simulink model "IEEE30_case"  (R2024b)
settings: Solver=FixedStepAuto  StartTime=0  StopTime=5  FixedStep=1e-7  RelTol=1e-3
values from neighbouring files (symbols this model uses):
  GFL_DFIG_7_C_bus = 0.08    [IEEE30_case_parameters.m]
  GFL_DFIG_7_D_mutual = 2.500000e+3    (= 2500)    [IEEE30_case_parameters.m]
  GFL_DFIG_7_f0 = 60    [IEEE30_case_parameters.m]
  GFL_DFIG_7_gPLLi = 3200    [IEEE30_case_parameters.m]
  GFL_DFIG_7_gPLLp = 650    [IEEE30_case_parameters.m]
  GFL_DFIG_7_H_WT = 0.4    [IEEE30_case_parameters.m]
  GFL_DFIG_7_Hg = 0.8    [IEEE30_case_parameters.m]
  GFL_DFIG_7_Igq_ref = 0    [IEEE30_case_parameters.m]
  GFL_DFIG_7_Ird_ref = 704.45696    [IEEE30_case_parameters.m]
  GFL_DFIG_7_KI_V = -300000    [IEEE30_case_parameters.m]
  GFL_DFIG_7_KP_V = -1000    [IEEE30_case_parameters.m]
  GFL_DFIG_7_Ksh = 1.254300e+4    (= 12543)    [IEEE30_case_parameters.m]
  GFL_DFIG_7_Lg = 0.000483    [IEEE30_case_parameters.m]
  GFL_DFIG_7_Lm_pu = 4    [IEEE30_case_parameters.m]
  GFL_DFIG_7_N = 100    [IEEE30_case_parameters.m]
  GFL_DFIG_7_p = 2    [IEEE30_case_parameters.m]
  GFL_DFIG_7_Pitch = 0    [IEEE30_case_parameters.m]
  GFL_DFIG_7_R = 44    [IEEE30_case_parameters.m]
  GFL_DFIG_7_Rg = 2.000000e-5    (= 2e-05)    [IEEE30_case_parameters.m]
  GFL_DFIG_7_rho = 1.225    [IEEE30_case_parameters.m]
  GFL_DFIG_7_rPLLi = 4500    [IEEE30_case_parameters.m]
  GFL_DFIG_7_rPLLp = 620    [IEEE30_case_parameters.m]
  GFL_DFIG_7_Rs_pu = 0.011    [IEEE30_case_parameters.m]
  GFL_DFIG_7_Sbase = 2.000000e+6    (= 2000000)    [IEEE30_case_parameters.m]
  GFL_DFIG_7_ugq_ref = 0    [IEEE30_case_parameters.m]
  GFL_DFIG_7_usd_ref = 0    [IEEE30_case_parameters.m]
  GFL_DFIG_7_Vbase = 690    [IEEE30_case_parameters.m]
  GFL_DFIG_7_Vdc_ref = 1200    [IEEE30_case_parameters.m]
  GFL_DFIG_7_wind = 12    [IEEE30_case_parameters.m]
  GFL_DFIG_7_wm_ref = 518.184209    [IEEE30_case_parameters.m]
  SG_D_13_D = 0.01056    [IEEE30_case_parameters.m]
  SG_D_13_EnableSaturation = 0    [IEEE30_case_parameters.m]
  SG_D_13_f0 = 60    [IEEE30_case_parameters.m]
  SG_D_13_H = 7.5    [IEEE30_case_parameters.m]
  SG_D_13_K_A = 20    [IEEE30_case_parameters.m]
  SG_D_13_K_E = 1.000000e+1    (= 10)    [IEEE30_case_parameters.m]
  SG_D_13_K_F = 2.363    [IEEE30_case_parameters.m]
  SG_D_13_K_s = 0.5    [IEEE30_case_parameters.m]
  SG_D_13_R_a = 0.001088    [IEEE30_case_parameters.m]
  SG_D_13_S_A = 1    [IEEE30_case_parameters.m]
  SG_D_13_S_B = 0.103    [IEEE30_case_parameters.m]
  SG_D_13_S_N = 10.659857    [IEEE30_case_parameters.m]
  SG_D_13_SpeedPara = 200    [IEEE30_case_parameters.m]
  SG_D_13_T_0 = 0.370163    [IEEE30_case_parameters.m]
  SG_D_13_T_1 = 0.3    [IEEE30_case_parameters.m]
  SG_D_13_T_2 = 0.05    [IEEE30_case_parameters.m]
  SG_D_13_T_3 = 0.02    [IEEE30_case_parameters.m]
  SG_D_13_T_4 = 0.005    [IEEE30_case_parameters.m]
  SG_D_13_T_A = 0.02    [IEEE30_case_parameters.m]
  SG_D_13_T_dd = 8.000000e+0    (= 8)    [IEEE30_case_parameters.m]
  SG_D_13_T_ddd = 0.04    [IEEE30_case_parameters.m]
  SG_D_13_T_E = 0.314    [IEEE30_case_parameters.m]
  SG_D_13_T_F = 0.35    [IEEE30_case_parameters.m]
  SG_D_13_T_qd = 0.8    [IEEE30_case_parameters.m]
  SG_D_13_T_qdd = 0.02    [IEEE30_case_parameters.m]
  SG_D_13_T_speed = 0.1    [IEEE30_case_parameters.m]
  SG_D_13_T_w = 0.5    [IEEE30_case_parameters.m]
  SG_D_13_V_ref = 1.696619    [IEEE30_case_parameters.m]
  SG_D_13_w_ref = 376.991118    [IEEE30_case_parameters.m]
  SG_D_13_x_d = 1.9    [IEEE30_case_parameters.m]
  SG_D_13_x_dd = 0.302    [IEEE30_case_parameters.m]
  SG_D_13_x_ddd = 0.204    [IEEE30_case_parameters.m]
  SG_D_13_x_l = 0.05    [IEEE30_case_parameters.m]
  SG_D_13_x_q = 1.3    [IEEE30_case_parameters.m]
  SG_D_13_x_qd = 0.5    [IEEE30_case_parameters.m]
  SG_D_13_x_qdd = 0.3    [IEEE30_case_parameters.m]
  SG_D_1_D = 0.01056    [IEEE30_case_parameters.m]
  SG_D_1_EnableSaturation = 0    [IEEE30_case_parameters.m]
  SG_D_1_f0 = 60    [IEEE30_case_parameters.m]
  SG_D_1_H = 7.5    [IEEE30_case_parameters.m]
  SG_D_1_K_A = 20    [IEEE30_case_parameters.m]
  SG_D_1_K_E = 1.000000e+1    (= 10)    [IEEE30_case_parameters.m]
  SG_D_1_K_F = 2.363    [IEEE30_case_parameters.m]
  SG_D_1_K_s = 0.5    [IEEE30_case_parameters.m]
  SG_D_1_R_a = 0.001088    [IEEE30_case_parameters.m]
  SG_D_1_S_A = 1    [IEEE30_case_parameters.m]
  SG_D_1_S_B = 0.103    [IEEE30_case_parameters.m]
  SG_D_1_S_N = 10.659857    [IEEE30_case_parameters.m]
  SG_D_1_SpeedPara = 200    [IEEE30_case_parameters.m]
  SG_D_1_T_0 = 0.259812    [IEEE30_case_parameters.m]
  SG_D_1_T_1 = 0.3    [IEEE30_case_parameters.m]
  SG_D_1_T_2 = 0.05    [IEEE30_case_parameters.m]
  SG_D_1_T_3 = 0.02    [IEEE30_case_parameters.m]
  SG_D_1_T_4 = 0.005    [IEEE30_case_parameters.m]
  SG_D_1_T_A = 0.02    [IEEE30_case_parameters.m]
  SG_D_1_T_dd = 8.000000e+0    (= 8)    [IEEE30_case_parameters.m]
  SG_D_1_T_ddd = 0.04    [IEEE30_case_parameters.m]
  SG_D_1_T_E = 0.314    [IEEE30_case_parameters.m]
  SG_D_1_T_F = 0.35    [IEEE30_case_parameters.m]
  SG_D_1_T_qd = 0.8    [IEEE30_case_parameters.m]
  SG_D_1_T_qdd = 0.02    [IEEE30_case_parameters.m]
  SG_D_1_T_speed = 0.1    [IEEE30_case_parameters.m]
  SG_D_1_T_w = 0.5    [IEEE30_case_parameters.m]
  SG_D_1_V_ref = 1.544107    [IEEE30_case_parameters.m]
  SG_D_1_w_ref = 376.991118    [IEEE30_case_parameters.m]
  SG_D_1_x_d = 1.9    [IEEE30_case_parameters.m]
  SG_D_1_x_dd = 0.302    [IEEE30_case_parameters.m]
  SG_D_1_x_ddd = 0.204    [IEEE30_case_parameters.m]
  SG_D_1_x_l = 0.05    [IEEE30_case_parameters.m]
  SG_D_1_x_q = 1.3    [IEEE30_case_parameters.m]
  SG_D_1_x_qd = 0.5    [IEEE30_case_parameters.m]
  SG_D_1_x_qdd = 0.3    [IEEE30_case_parameters.m]
  SG_D_22_D = 0.01056    [IEEE30_case_parameters.m]
  SG_D_22_EnableSaturation = 0    [IEEE30_case_parameters.m]
  SG_D_22_f0 = 60    [IEEE30_case_parameters.m]
  SG_D_22_H = 7.5    [IEEE30_case_parameters.m]
  SG_D_22_K_A = 20    [IEEE30_case_parameters.m]
  SG_D_22_K_E = 1.000000e+1    (= 10)    [IEEE30_case_parameters.m]
  SG_D_22_K_F = 2.363    [IEEE30_case_parameters.m]
  SG_D_22_K_s = 0.5    [IEEE30_case_parameters.m]
  SG_D_22_R_a = 0.001088    [IEEE30_case_parameters.m]
  SG_D_22_S_A = 1    [IEEE30_case_parameters.m]
  SG_D_22_S_B = 0.103    [IEEE30_case_parameters.m]
  SG_D_22_S_N = 10.659857    [IEEE30_case_parameters.m]
  SG_D_22_SpeedPara = 200    [IEEE30_case_parameters.m]
  SG_D_22_T_0 = 0.216121    [IEEE30_case_parameters.m]
  SG_D_22_T_1 = 0.3    [IEEE30_case_parameters.m]
  SG_D_22_T_2 = 0.05    [IEEE30_case_parameters.m]
  SG_D_22_T_3 = 0.02    [IEEE30_case_parameters.m]
  SG_D_22_T_4 = 0.005    [IEEE30_case_parameters.m]
  ... (+126 more)
(part 10 of 27)

== system IEEE30_case/AC_1/d_vq_bus_23_block ==
  note: d_vq_bus_23 in IEEE30_case
      | $37699111.8430775\,\mathrm{iq}_{\mathrm{bus},23}-376.991118430775\,\mathrm{vd}_{\mathrm{bus},23}$
      | Automatically generated on 2025-11-01 18:40:01 .
  Alge_iq_bus_23_4fd9f : Inport
  State_vd_bus_23_43c98 : Inport  Port=2
  Constant_376.991118430775_89ee7 : Constant  Value=376.991118430775
  Constant_37699111.8430775_5a930 : Constant  Value=37699111.8430775
  Product_5f7b2 : Product
  Product_6759d : Product
  Subtract_d8bec : Sum  Inputs=+-
  Blockout_d_vq_bus_23_b171c : Outport
  wires:
  Constant_37699111.8430775_5a930/1 -> Product_5f7b2/1
  Alge_iq_bus_23_4fd9f/1 -> Product_5f7b2/2
  Product_6759d/1 -> Subtract_d8bec/2
  State_vd_bus_23_43c98/1 -> Product_6759d/2
  Constant_376.991118430775_89ee7/1 -> Product_6759d/1
  Product_5f7b2/1 -> Subtract_d8bec/1
  Subtract_d8bec/1 -> Blockout_d_vq_bus_23_b171c/1

== system IEEE30_case/AC_1/d_vq_bus_24_block ==
  note: d_vq_bus_24 in IEEE30_case
      | $942477.796076938\,\mathrm{iq}_{\mathrm{bus},24}-376.991118430775\,\mathrm{vd}_{\mathrm{bus},24}$
      | Automatically generated on 2025-11-01 18:40:03 .
  Alge_iq_bus_24_0b825 : Inport
  State_vd_bus_24_b47e7 : Inport  Port=2
  Constant_376.991118430775_6b77a : Constant  Value=376.991118430775
  Constant_942477.796076938_b7520 : Constant  Value=942477.796076938
  Product_085e8 : Product
  Product_cc19f : Product
  Subtract_a05e3 : Sum  Inputs=+-
  Blockout_d_vq_bus_24_2859e : Outport
  wires:
  State_vd_bus_24_b47e7/1 -> Product_085e8/2
  Constant_942477.796076938_b7520/1 -> Product_cc19f/1
  Product_085e8/1 -> Subtract_a05e3/2
  Constant_376.991118430775_6b77a/1 -> Product_085e8/1
  Alge_iq_bus_24_0b825/1 -> Product_cc19f/2
  Product_cc19f/1 -> Subtract_a05e3/1
  Subtract_a05e3/1 -> Blockout_d_vq_bus_24_2859e/1

== system IEEE30_case/AC_1/d_vq_bus_25_block ==
  note: d_vq_bus_25 in IEEE30_case
      | $37699111.8430775\,\mathrm{iq}_{\mathrm{bus},25}-376.991118430775\,\mathrm{vd}_{\mathrm{bus},25}$
      | Automatically generated on 2025-11-01 18:40:05 .
  Alge_iq_bus_25_b52f0 : Inport
  State_vd_bus_25_5727a : Inport  Port=2
  Constant_376.991118430775_a3e2e : Constant  Value=376.991118430775
  Constant_37699111.8430775_b0c0a : Constant  Value=37699111.8430775
  Product_022ff : Product
  Product_2edfc : Product
  Subtract_ce7e6 : Sum  Inputs=+-
  Blockout_d_vq_bus_25_e403d : Outport
  wires:
  Alge_iq_bus_25_b52f0/1 -> Product_2edfc/2
  Constant_37699111.8430775_b0c0a/1 -> Product_2edfc/1
  Product_022ff/1 -> Subtract_ce7e6/2
  Constant_376.991118430775_a3e2e/1 -> Product_022ff/1
  State_vd_bus_25_5727a/1 -> Product_022ff/2
  Product_2edfc/1 -> Subtract_ce7e6/1
  Subtract_ce7e6/1 -> Blockout_d_vq_bus_25_e403d/1

== system IEEE30_case/AC_1/d_vq_bus_26_block ==
  note: d_vq_bus_26 in IEEE30_case
      | $37699111.8430775\,\mathrm{iq}_{\mathrm{bus},26}-376.991118430775\,\mathrm{vd}_{\mathrm{bus},26}$
      | Automatically generated on 2025-11-01 18:40:07 .
  Alge_iq_bus_26_172b0 : Inport
  State_vd_bus_26_21468 : Inport  Port=2
  Constant_376.991118430775_b7844 : Constant  Value=376.991118430775
  Constant_37699111.8430775_77cc8 : Constant  Value=37699111.8430775
  Product_15b09 : Product
  Product_a4d83 : Product
  Subtract_d1cbb : Sum  Inputs=+-
  Blockout_d_vq_bus_26_2e68a : Outport
  wires:
  Subtract_d1cbb/1 -> Blockout_d_vq_bus_26_2e68a/1
  Constant_37699111.8430775_77cc8/1 -> Product_a4d83/1
  Alge_iq_bus_26_172b0/1 -> Product_a4d83/2
  Constant_376.991118430775_b7844/1 -> Product_15b09/1
  Product_a4d83/1 -> Subtract_d1cbb/1
  State_vd_bus_26_21468/1 -> Product_15b09/2
  Product_15b09/1 -> Subtract_d1cbb/2

== system IEEE30_case/AC_1/d_vq_bus_27_block ==
  note: d_vq_bus_27 in IEEE30_case
      | $37699111.8430775\,\mathrm{iq}_{\mathrm{bus},27}-376.991118430775\,\mathrm{vd}_{\mathrm{bus},27}$
      | Automatically generated on 2025-11-01 18:40:08 .
  Alge_iq_bus_27_548e5 : Inport
  State_vd_bus_27_e355a : Inport  Port=2
  Constant_376.991118430775_3be52 : Constant  Value=376.991118430775
  Constant_37699111.8430775_fd80b : Constant  Value=37699111.8430775
  Product_a7865 : Product
  Product_b7592 : Product
  Subtract_05554 : Sum  Inputs=+-
  Blockout_d_vq_bus_27_9b6db : Outport
  wires:
  Subtract_05554/1 -> Blockout_d_vq_bus_27_9b6db/1
  Constant_37699111.8430775_fd80b/1 -> Product_b7592/1
  Alge_iq_bus_27_548e5/1 -> Product_b7592/2
  Product_a7865/1 -> Subtract_05554/2
  Constant_376.991118430775_3be52/1 -> Product_a7865/1
  Product_b7592/1 -> Subtract_05554/1
  State_vd_bus_27_e355a/1 -> Product_a7865/2

== system IEEE30_case/AC_1/d_vq_bus_28_block ==
  note: d_vq_bus_28 in IEEE30_case
      | $25132.7412287183\,\mathrm{iq}_{\mathrm{bus},28}-376.991118430775\,\mathrm{vd}_{\mathrm{bus},28}$
      | Automatically generated on 2025-11-01 18:40:10 .
  Alge_iq_bus_28_e3380 : Inport
  State_vd_bus_28_5e73c : Inport  Port=2
  Constant_25132.7412287183_edff6 : Constant  Value=25132.7412287183
  Constant_376.991118430775_78daa : Constant  Value=376.991118430775
  Product_1f4c4 : Product
  Product_9eeee : Product
  Subtract_e11d4 : Sum  Inputs=+-
  Blockout_d_vq_bus_28_fc78f : Outport
  wires:
  Constant_25132.7412287183_edff6/1 -> Product_1f4c4/1
  Alge_iq_bus_28_e3380/1 -> Product_1f4c4/2
  Product_9eeee/1 -> Subtract_e11d4/2
  Constant_376.991118430775_78daa/1 -> Product_9eeee/1
  Product_1f4c4/1 -> Subtract_e11d4/1
  State_vd_bus_28_5e73c/1 -> Product_9eeee/2
  Subtract_e11d4/1 -> Blockout_d_vq_bus_28_fc78f/1

== system IEEE30_case/AC_1/d_vq_bus_29_block ==
  note: d_vq_bus_29 in IEEE30_case
      | $37699111.8430775\,\mathrm{iq}_{\mathrm{bus},29}-376.991118430775\,\mathrm{vd}_{\mathrm{bus},29}$
      | Automatically generated on 2025-11-01 18:40:12 .
  Alge_iq_bus_29_a773e : Inport
  State_vd_bus_29_8221e : Inport  Port=2
  Constant_376.991118430775_ce99e : Constant  Value=376.991118430775
  Constant_37699111.8430775_7e507 : Constant  Value=37699111.8430775
  Product_4bf07 : Product
  Product_e159a : Product
  Subtract_59131 : Sum  Inputs=+-
  Blockout_d_vq_bus_29_9ca95 : Outport
  wires:
  Subtract_59131/1 -> Blockout_d_vq_bus_29_9ca95/1
  Constant_37699111.8430775_7e507/1 -> Product_4bf07/1
  Alge_iq_bus_29_a773e/1 -> Product_4bf07/2
  Product_e159a/1 -> Subtract_59131/2
  Constant_376.991118430775_ce99e/1 -> Product_e159a/1
  Product_4bf07/1 -> Subtract_59131/1
  State_vd_bus_29_8221e/1 -> Product_e159a/2

== system IEEE30_case/AC_1/d_vq_bus_2_block ==
  note: d_vq_bus_2 in IEEE30_case
      | $8377.58040957278\,\mathrm{iq}_{\mathrm{bus},2}-376.991118430775\,\mathrm{vd}_{\mathrm{bus},2}$
      | Automatically generated on 2025-11-01 18:39:26 .
  Alge_iq_bus_2_6cf64 : Inport
  State_vd_bus_2_c8ab9 : Inport  Port=2
  Constant_376.991118430775_774b2 : Constant  Value=376.991118430775
  Constant_8377.58040957278_cfb02 : Constant  Value=8377.58040957278
  Product_7f39e : Product
  Product_d1afe : Product
  Subtract_105ce : Sum  Inputs=+-
  Blockout_d_vq_bus_2_d5528 : Outport
  wires:
  Subtract_105ce/1 -> Blockout_d_vq_bus_2_d5528/1
  Constant_8377.58040957278_cfb02/1 -> Product_7f39e/1
  Alge_iq_bus_2_6cf64/1 -> Product_7f39e/2
  Constant_376.991118430775_774b2/1 -> Product_d1afe/1
  Product_7f39e/1 -> Subtract_105ce/1
  State_vd_bus_2_c8ab9/1 -> Product_d1afe/2
  Product_d1afe/1 -> Subtract_105ce/2

== system IEEE30_case/AC_1/d_vq_bus_30_block ==
  note: d_vq_bus_30 in IEEE30_case
      | $37699111.8430775\,\mathrm{iq}_{\mathrm{bus},30}-376.991118430775\,\mathrm{vd}_{\mathrm{bus},30}$
      | Automatically generated on 2025-11-01 18:40:13 .
  Alge_iq_bus_30_b84d2 : Inport
  State_vd_bus_30_536bd : Inport  Port=2
  Constant_376.991118430775_6c92f : Constant  Value=376.991118430775
  Constant_37699111.8430775_51ba2 : Constant  Value=37699111.8430775
  Product_8ec72 : Product
  Product_a9806 : Product
  Subtract_97059 : Sum  Inputs=+-
  Blockout_d_vq_bus_30_e3d22 : Outport
  wires:
  Subtract_97059/1 -> Blockout_d_vq_bus_30_e3d22/1
  Constant_37699111.8430775_51ba2/1 -> Product_a9806/1
  Alge_iq_bus_30_b84d2/1 -> Product_a9806/2
  Constant_376.991118430775_6c92f/1 -> Product_8ec72/1
  Product_a9806/1 -> Subtract_97059/1
  State_vd_bus_30_536bd/1 -> Product_8ec72/2
  Product_8ec72/1 -> Subtract_97059/2

== system IEEE30_case/AC_1/d_vq_bus_3_block ==
  note: d_vq_bus_3 in IEEE30_case
      | $37699.1118430775\,\mathrm{iq}_{\mathrm{bus},3}-376.991118430775\,\mathrm{vd}_{\mathrm{bus},3}$
      | Automatically generated on 2025-11-01 18:39:27 .
  Alge_iq_bus_3_cb5cd : Inport
  State_vd_bus_3_2475d : Inport  Port=2
  Constant_376.991118430775_40eb7 : Constant  Value=376.991118430775
  Constant_37699.1118430775_dedd8 : Constant  Value=37699.1118430775
  Product_a5528 : Product
  Product_bea63 : Product
  Subtract_577e7 : Sum  Inputs=+-
  Blockout_d_vq_bus_3_10f19 : Outport
  wires:
  Subtract_577e7/1 -> Blockout_d_vq_bus_3_10f19/1
  Constant_37699.1118430775_dedd8/1 -> Product_a5528/1
  Alge_iq_bus_3_cb5cd/1 -> Product_a5528/2
  Product_bea63/1 -> Subtract_577e7/2
  Constant_376.991118430775_40eb7/1 -> Product_bea63/1
  Product_a5528/1 -> Subtract_577e7/1
  State_vd_bus_3_2475d/1 -> Product_bea63/2

== system IEEE30_case/AC_1/d_vq_bus_4_block ==
  note: d_vq_bus_4 in IEEE30_case
      | $37699.1118430775\,\mathrm{iq}_{\mathrm{bus},4}-376.991118430775\,\mathrm{vd}_{\mathrm{bus},4}$
      | Automatically generated on 2025-11-01 18:39:29 .
  Alge_iq_bus_4_edea5 : Inport
  State_vd_bus_4_783ad : Inport  Port=2
  Constant_376.991118430775_7c085 : Constant  Value=376.991118430775
  Constant_37699.1118430775_1ff83 : Constant  Value=37699.1118430775
  Product_afb80 : Product
  Product_bbdae : Product
  Subtract_ff271 : Sum  Inputs=+-
  Blockout_d_vq_bus_4_757f0 : Outport
  wires:
  Constant_37699.1118430775_1ff83/1 -> Product_afb80/1
  Alge_iq_bus_4_edea5/1 -> Product_afb80/2
  Product_bbdae/1 -> Subtract_ff271/2
  Constant_376.991118430775_7c085/1 -> Product_bbdae/1
  Product_afb80/1 -> Subtract_ff271/1
  State_vd_bus_4_783ad/1 -> Product_bbdae/2
  Subtract_ff271/1 -> Blockout_d_vq_bus_4_757f0/1

== system IEEE30_case/AC_1/d_vq_bus_5_block ==
  note: d_vq_bus_5 in IEEE30_case
      | $22307.1667710518\,\mathrm{iq}_{\mathrm{bus},5}-376.991118430775\,\mathrm{vd}_{\mathrm{bus},5}$
      | Automatically generated on 2025-11-01 18:39:31 .
  Alge_iq_bus_5_20adf : Inport
  State_vd_bus_5_28f77 : Inport  Port=2
  Constant_22307.1667710518_b913d : Constant  Value=22307.1667710518
  Constant_376.991118430775_7861f : Constant  Value=376.991118430775
  Product_25fa6 : Product
  Product_cf06c : Product
  Subtract_2168d : Sum  Inputs=+-
  Blockout_d_vq_bus_5_f1f0c : Outport
  wires:
  Constant_22307.1667710518_b913d/1 -> Product_25fa6/1
  Product_cf06c/1 -> Subtract_2168d/2
  Constant_376.991118430775_7861f/1 -> Product_cf06c/1
  Alge_iq_bus_5_20adf/1 -> Product_25fa6/2
  State_vd_bus_5_28f77/1 -> Product_cf06c/2
  Product_25fa6/1 -> Subtract_2168d/1
  Subtract_2168d/1 -> Blockout_d_vq_bus_5_f1f0c/1

== system IEEE30_case/AC_1/d_vq_bus_6_block ==
  note: d_vq_bus_6 in IEEE30_case
      | $18849.5559215388\,\mathrm{iq}_{\mathrm{bus},6}-376.991118430775\,\mathrm{vd}_{\mathrm{bus},6}$
      | Automatically generated on 2025-11-01 18:39:32 .
  Alge_iq_bus_6_8f458 : Inport
  State_vd_bus_6_1a151 : Inport  Port=2
  Constant_18849.5559215388_854b2 : Constant  Value=18849.5559215388
  Constant_376.991118430775_77bfe : Constant  Value=376.991118430775
  Product_ad02e : Product
  Product_e2853 : Product
  Subtract_ccaa3 : Sum  Inputs=+-
  Blockout_d_vq_bus_6_ac6cf : Outport
  wires:
  Constant_18849.5559215388_854b2/1 -> Product_ad02e/1
  Product_e2853/1 -> Subtract_ccaa3/2
  Alge_iq_bus_6_8f458/1 -> Product_ad02e/2
  Constant_376.991118430775_77bfe/1 -> Product_e2853/1
  State_vd_bus_6_1a151/1 -> Product_e2853/2
  Product_ad02e/1 -> Subtract_ccaa3/1
  Subtract_ccaa3/1 -> Blockout_d_vq_bus_6_ac6cf/1

== system IEEE30_case/AC_1/d_vq_bus_7_block ==
  note: d_vq_bus_7 in IEEE30_case
      | $37699.1118430775\,\mathrm{iq}_{\mathrm{bus},7}-376.991118430775\,\mathrm{vd}_{\mathrm{bus},7}$
      | Automatically generated on 2025-11-01 18:39:34 .
  Alge_iq_bus_7_86528 : Inport
  State_vd_bus_7_0bd1f : Inport  Port=2
  Constant_376.991118430775_95f94 : Constant  Value=376.991118430775
  Constant_37699.1118430775_46c75 : Constant  Value=37699.1118430775
  Product_8c587 : Product
  Product_cc660 : Product
  Subtract_38f8c : Sum  Inputs=+-
  Blockout_d_vq_bus_7_71b97 : Outport
  wires:
  Subtract_38f8c/1 -> Blockout_d_vq_bus_7_71b97/1
  Constant_37699.1118430775_46c75/1 -> Product_cc660/1
  Alge_iq_bus_7_86528/1 -> Product_cc660/2
  Product_8c587/1 -> Subtract_38f8c/2
  Constant_376.991118430775_95f94/1 -> Product_8c587/1
  Product_cc660/1 -> Subtract_38f8c/1
  State_vd_bus_7_0bd1f/1 -> Product_8c587/2

== system IEEE30_case/AC_1/d_vq_bus_8_block ==
  note: d_vq_bus_8 in IEEE30_case
      | $37699.1118430775\,\mathrm{iq}_{\mathrm{bus},8}-376.991118430775\,\mathrm{vd}_{\mathrm{bus},8}$
      | Automatically generated on 2025-11-01 18:39:36 .
  Alge_iq_bus_8_bb8a6 : Inport
  State_vd_bus_8_8cd22 : Inport  Port=2
  Constant_376.991118430775_aa994 : Constant  Value=376.991118430775
  Constant_37699.1118430775_3c9b2 : Constant  Value=37699.1118430775
  Product_1950e : Product
  Product_8773e : Product
  Subtract_0dd82 : Sum  Inputs=+-
  Blockout_d_vq_bus_8_7917f : Outport
  wires:
  Constant_37699.1118430775_3c9b2/1 -> Product_1950e/1
  Alge_iq_bus_8_bb8a6/1 -> Product_1950e/2
  Product_8773e/1 -> Subtract_0dd82/2
  Constant_376.991118430775_aa994/1 -> Product_8773e/1
  Product_1950e/1 -> Subtract_0dd82/1
  State_vd_bus_8_8cd22/1 -> Product_8773e/2
  Subtract_0dd82/1 -> Blockout_d_vq_bus_8_7917f/1

== system IEEE30_case/AC_1/d_vq_bus_9_block ==
  note: d_vq_bus_9 in IEEE30_case
      | $37699111.8430775\,\mathrm{iq}_{\mathrm{bus},9}-376.991118430775\,\mathrm{vd}_{\mathrm{bus},9}$
      | Automatically generated on 2025-11-01 18:39:37 .
  Alge_iq_bus_9_8054c : Inport
  State_vd_bus_9_08774 : Inport  Port=2
  Constant_376.991118430775_3b7d3 : Constant  Value=376.991118430775
  Constant_37699111.8430775_a1b9d : Constant  Value=37699111.8430775
  Product_85a06 : Product
  Product_e292a : Product
  Subtract_b525b : Sum  Inputs=+-
  Blockout_d_vq_bus_9_087a9 : Outport
  wires:
  Subtract_b525b/1 -> Blockout_d_vq_bus_9_087a9/1
  Constant_37699111.8430775_a1b9d/1 -> Product_e292a/1
  Alge_iq_bus_9_8054c/1 -> Product_e292a/2
  Product_85a06/1 -> Subtract_b525b/2
  Constant_376.991118430775_3b7d3/1 -> Product_85a06/1
  Product_e292a/1 -> Subtract_b525b/1
  State_vd_bus_9_08774/1 -> Product_85a06/2

== system IEEE30_case/AC_1/id_bus_10_block ==
  note: id_bus_10 in IEEE30_case
      | $\mathrm{id}_{\mathrm{line},6,10}-\mathrm{id}_{\mathrm{load},10}+\mathrm{id}_{\mathrm{line},9,10}-\mathrm{id}_{\mathrm{line},10,17}-\mathrm{id}_{\mathrm{line},10,20}-\mathrm{id}_{\mathrm{line},10,21}-\mathrm{id}_{\mathrm{line},10,22}$
      | Automatically generated on 2025-11-01 18:42:51 .
  State_id_load_10_705f8 : Inport
  State_id_line_6_10_65dc9 : Inport  Port=2
  State_id_line_9_10_7013c : Inport  Port=3
  State_id_line_10_17_ef9ff : Inport  Port=4
  State_id_line_10_20_18f02 : Inport  Port=5
  State_id_line_10_21_c8fce : Inport  Port=6
  State_id_line_10_22_301e1 : Inport  Port=7
  Add_81d1d : Sum
  Add_d7f77 : Sum
  Constant_-1_c0d8a : Constant  Value=-1
  Product_b469d : Product
  Subtract_5d409 : Sum  Inputs=+-
  Subtract_9e640 : Sum  Inputs=+-
  Subtract_a236b : Sum  Inputs=+-
  Subtract_d925d : Sum  Inputs=+-
  Blockout_id_bus_10_f7cfc : Outport
  wires:
  Constant_-1_c0d8a/1 -> Product_b469d/1
  Product_b469d/1 -> Add_d7f77/1
  Add_d7f77/1 -> Add_81d1d/1
  Add_81d1d/1 -> Subtract_a236b/1
  State_id_load_10_705f8/1 -> Product_b469d/2
  State_id_line_6_10_65dc9/1 -> Add_d7f77/2
  State_id_line_10_17_ef9ff/1 -> Subtract_a236b/2
  State_id_line_9_10_7013c/1 -> Add_81d1d/2
  Subtract_5d409/1 -> Subtract_d925d/1
  Subtract_a236b/1 -> Subtract_5d409/1
  State_id_line_10_20_18f02/1 -> Subtract_5d409/2
  State_id_line_10_21_c8fce/1 -> Subtract_d925d/2
  State_id_line_10_22_301e1/1 -> Subtract_9e640/2
  Subtract_d925d/1 -> Subtract_9e640/1
  Subtract_9e640/1 -> Blockout_id_bus_10_f7cfc/1

== system IEEE30_case/AC_1/id_bus_11_block ==
  note: id_bus_11 in IEEE30_case
      | $\mathrm{id}_{\mathrm{line},9,11}$
      | Automatically generated on 2025-11-01 18:42:52 .
  State_id_line_9_11_37f59 : Inport
  Blockout_id_bus_11_04e0f : Outport
  wires:
  State_id_line_9_11_37f59/1 -> Blockout_id_bus_11_04e0f/1

== system IEEE30_case/AC_1/id_bus_12_block ==
  note: id_bus_12 in IEEE30_case
      | $\mathrm{id}_{\mathrm{line},4,12}-\mathrm{id}_{\mathrm{load},12}-\mathrm{id}_{\mathrm{line},12,13}-\mathrm{id}_{\mathrm{line},12,14}-\mathrm{id}_{\mathrm{line},12,15}-\mathrm{id}_{\mathrm{line},12,16}$
      | Automatically generated on 2025-11-01 18:42:54 .
  State_id_load_12_8eb9c : Inport
  State_id_line_4_12_8182e : Inport  Port=2
  State_id_line_12_13_02bcf : Inport  Port=3
  State_id_line_12_14_017fa : Inport  Port=4
  State_id_line_12_15_e30db : Inport  Port=5
  State_id_line_12_16_2f396 : Inport  Port=6
  Add_340d6 : Sum
  Constant_-1_6c20b : Constant  Value=-1
  Product_d81ab : Product
  Subtract_4b682 : Sum  Inputs=+-
  Subtract_956ec : Sum  Inputs=+-
  Subtract_d4719 : Sum  Inputs=+-
  Subtract_d9b2f : Sum  Inputs=+-
  Blockout_id_bus_12_a7f7d : Outport
  wires:
  Constant_-1_6c20b/1 -> Product_d81ab/1
  Product_d81ab/1 -> Add_340d6/1
  Add_340d6/1 -> Subtract_956ec/1
  State_id_line_4_12_8182e/1 -> Add_340d6/2
  State_id_load_12_8eb9c/1 -> Product_d81ab/2
  Subtract_4b682/1 -> Subtract_d4719/1
  Subtract_956ec/1 -> Subtract_4b682/1
  State_id_line_12_13_02bcf/1 -> Subtract_956ec/2
  State_id_line_12_14_017fa/1 -> Subtract_4b682/2
  State_id_line_12_15_e30db/1 -> Subtract_d4719/2
  Subtract_d4719/1 -> Subtract_d9b2f/1
  State_id_line_12_16_2f396/1 -> Subtract_d9b2f/2
  Subtract_d9b2f/1 -> Blockout_id_bus_12_a7f7d/1

== system IEEE30_case/AC_1/id_bus_13_block ==
  note: id_bus_13 in IEEE30_case
      | $\mathrm{id}_{\mathrm{SG},D,13}+\mathrm{id}_{\mathrm{line},12,13}$
      | Automatically generated on 2025-11-01 18:42:57 .
  Input_id_SG_D_13_a3cac : Inport
  State_id_line_12_13_e1ea8 : Inport  Port=2
  Add_1f282 : Sum
  Blockout_id_bus_13_e8139 : Outport
  wires:
  Add_1f282/1 -> Blockout_id_bus_13_e8139/1
  State_id_line_12_13_e1ea8/1 -> Add_1f282/2
  Input_id_SG_D_13_a3cac/1 -> Add_1f282/1

== system IEEE30_case/AC_1/id_bus_14_block ==
  note: id_bus_14 in IEEE30_case
      | $\mathrm{id}_{\mathrm{line},12,14}-\mathrm{id}_{\mathrm{load},14}-\mathrm{id}_{\mathrm{line},14,15}$
      | Automatically generated on 2025-11-01 18:42:58 .
  State_id_load_14_8acb6 : Inport
  State_id_line_12_14_e86dc : Inport  Port=2
  State_id_line_14_15_8760d : Inport  Port=3
  Add_4b372 : Sum
  Constant_-1_29924 : Constant  Value=-1
  Product_0535b : Product
  Subtract_f026d : Sum  Inputs=+-
  Blockout_id_bus_14_a7723 : Outport
  wires:
  Product_0535b/1 -> Add_4b372/1
  Constant_-1_29924/1 -> Product_0535b/1
  Add_4b372/1 -> Subtract_f026d/1
  State_id_line_12_14_e86dc/1 -> Add_4b372/2
  State_id_load_14_8acb6/1 -> Product_0535b/2
  State_id_line_14_15_8760d/1 -> Subtract_f026d/2
  Subtract_f026d/1 -> Blockout_id_bus_14_a7723/1

== system IEEE30_case/AC_1/id_bus_15_block ==
  note: id_bus_15 in IEEE30_case
      | $\mathrm{id}_{\mathrm{line},12,15}-\mathrm{id}_{\mathrm{load},15}+\mathrm{id}_{\mathrm{line},14,15}-\mathrm{id}_{\mathrm{line},15,18}-\mathrm{id}_{\mathrm{line},15,23}$
      | Automatically generated on 2025-11-01 18:43:00 .
  State_id_load_15_060ab : Inport
  State_id_line_12_15_8e417 : Inport  Port=2
  State_id_line_14_15_22f97 : Inport  Port=3
  State_id_line_15_18_9837d : Inport  Port=4
  State_id_line_15_23_df0bc : Inport  Port=5
  Add_c531c : Sum
  Add_d2721 : Sum
  Constant_-1_33c67 : Constant  Value=-1
  Product_a587d : Product
  Subtract_6212d : Sum  Inputs=+-
  Subtract_7f898 : Sum  Inputs=+-
  Blockout_id_bus_15_03e1f : Outport
  wires:
  Constant_-1_33c67/1 -> Product_a587d/1
  Product_a587d/1 -> Add_c531c/1
  State_id_line_12_15_8e417/1 -> Add_c531c/2
  State_id_load_15_060ab/1 -> Product_a587d/2
  Add_c531c/1 -> Add_d2721/1
  Add_d2721/1 -> Subtract_6212d/1
  State_id_line_15_18_9837d/1 -> Subtract_6212d/2
  State_id_line_14_15_22f97/1 -> Add_d2721/2
  Subtract_6212d/1 -> Subtract_7f898/1
  State_id_line_15_23_df0bc/1 -> Subtract_7f898/2
  Subtract_7f898/1 -> Blockout_id_bus_15_03e1f/1

== system IEEE30_case/AC_1/id_bus_16_block ==
  note: id_bus_16 in IEEE30_case
      | $\mathrm{id}_{\mathrm{line},12,16}-\mathrm{id}_{\mathrm{load},16}-\mathrm{id}_{\mathrm{line},16,17}$
      | Automatically generated on 2025-11-01 18:43:02 .
  State_id_load_16_85ef4 : Inport
  State_id_line_12_16_31af9 : Inport  Port=2
  State_id_line_16_17_d7b9d : Inport  Port=3
  Add_c2788 : Sum
  Constant_-1_e4b07 : Constant  Value=-1
  Product_aea95 : Product
  Subtract_c106b : Sum  Inputs=+-
  Blockout_id_bus_16_3e58c : Outport
  wires:
  Constant_-1_e4b07/1 -> Product_aea95/1
  State_id_line_12_16_31af9/1 -> Add_c2788/2
  State_id_load_16_85ef4/1 -> Product_aea95/2
  Product_aea95/1 -> Add_c2788/1
  Subtract_c106b/1 -> Blockout_id_bus_16_3e58c/1
  Add_c2788/1 -> Subtract_c106b/1
  State_id_line_16_17_d7b9d/1 -> Subtract_c106b/2

== system IEEE30_case/AC_1/id_bus_17_block ==
  note: id_bus_17 in IEEE30_case
      | $\mathrm{id}_{\mathrm{line},10,17}-\mathrm{id}_{\mathrm{load},17}+\mathrm{id}_{\mathrm{line},16,17}$
      | Automatically generated on 2025-11-01 18:43:04 .
  State_id_load_17_98f31 : Inport
  State_id_line_10_17_3b6f4 : Inport  Port=2
  State_id_line_16_17_e2e89 : Inport  Port=3
  Add_4d1b5 : Sum
  Add_d5a9b : Sum
  Constant_-1_d3cb0 : Constant  Value=-1
  Product_e65a9 : Product
  Blockout_id_bus_17_5f54e : Outport
  wires:
  Product_e65a9/1 -> Add_d5a9b/1
  Constant_-1_d3cb0/1 -> Product_e65a9/1
  Add_d5a9b/1 -> Add_4d1b5/1
  State_id_line_10_17_3b6f4/1 -> Add_d5a9b/2
  State_id_load_17_98f31/1 -> Product_e65a9/2
  State_id_line_16_17_e2e89/1 -> Add_4d1b5/2
  Add_4d1b5/1 -> Blockout_id_bus_17_5f54e/1

== system IEEE30_case/AC_1/id_bus_18_block ==
  note: id_bus_18 in IEEE30_case
      | $\mathrm{id}_{\mathrm{line},15,18}-\mathrm{id}_{\mathrm{load},18}-\mathrm{id}_{\mathrm{line},18,19}$
      | Automatically generated on 2025-11-01 18:43:05 .
  State_id_load_18_b6089 : Inport
  State_id_line_15_18_185de : Inport  Port=2
  State_id_line_18_19_1fd25 : Inport  Port=3
  Add_02070 : Sum
  Constant_-1_09ca4 : Constant  Value=-1
  Product_47eef : Product
  Subtract_a4093 : Sum  Inputs=+-
  Blockout_id_bus_18_f6aba : Outport
  wires:
  Subtract_a4093/1 -> Blockout_id_bus_18_f6aba/1
  Product_47eef/1 -> Add_02070/1
  Constant_-1_09ca4/1 -> Product_47eef/1
  State_id_load_18_b6089/1 -> Product_47eef/2
  Add_02070/1 -> Subtract_a4093/1
  State_id_line_15_18_185de/1 -> Add_02070/2
  State_id_line_18_19_1fd25/1 -> Subtract_a4093/2

== system IEEE30_case/AC_1/id_bus_19_block ==
  note: id_bus_19 in IEEE30_case
      | $\mathrm{id}_{\mathrm{line},18,19}-\mathrm{id}_{\mathrm{load},19}-\mathrm{id}_{\mathrm{line},19,20}$
      | Automatically generated on 2025-11-01 18:43:07 .
  State_id_load_19_6dd0b : Inport
  State_id_line_18_19_4e3a3 : Inport  Port=2
  State_id_line_19_20_f791c : Inport  Port=3
  Add_1b5aa : Sum
  Constant_-1_3ab29 : Constant  Value=-1
  Product_b6dd6 : Product
  Subtract_f828e : Sum  Inputs=+-
  Blockout_id_bus_19_c959d : Outport
  wires:
  State_id_line_19_20_f791c/1 -> Subtract_f828e/2
  State_id_line_18_19_4e3a3/1 -> Add_1b5aa/2
  Constant_-1_3ab29/1 -> Product_b6dd6/1
  State_id_load_19_6dd0b/1 -> Product_b6dd6/2
  Product_b6dd6/1 -> Add_1b5aa/1
  Add_1b5aa/1 -> Subtract_f828e/1
  Subtract_f828e/1 -> Blockout_id_bus_19_c959d/1

== system IEEE30_case/AC_1/id_bus_1_block ==
  note: id_bus_1 in IEEE30_case
      | $\mathrm{id}_{\mathrm{SG},D,1}-\mathrm{id}_{\mathrm{line},1,2}-\mathrm{id}_{\mathrm{line},1,3}$
      | Automatically generated on 2025-11-01 18:42:33 .
  Input_id_SG_D_1_df3b6 : Inport
  State_id_line_1_2_dfc68 : Inport  Port=2
  State_id_line_1_3_6e2c0 : Inport  Port=3
  Subtract_07953 : Sum  Inputs=+-
  Subtract_3984d : Sum  Inputs=+-
  Blockout_id_bus_1_c8a02 : Outport
  wires:
  Input_id_SG_D_1_df3b6/1 -> Subtract_3984d/1
  State_id_line_1_2_dfc68/1 -> Subtract_3984d/2
  Subtract_3984d/1 -> Subtract_07953/1
  State_id_line_1_3_6e2c0/1 -> Subtract_07953/2
  Subtract_07953/1 -> Blockout_id_bus_1_c8a02/1

== system IEEE30_case/AC_1/id_bus_20_block ==
  note: id_bus_20 in IEEE30_case
      | $\mathrm{id}_{\mathrm{line},10,20}-\mathrm{id}_{\mathrm{load},20}+\mathrm{id}_{\mathrm{line},19,20}$
      | Automatically generated on 2025-11-01 18:43:09 .
  State_id_load_20_3e20a : Inport
  State_id_line_10_20_7e98a : Inport  Port=2
  State_id_line_19_20_ee948 : Inport  Port=3
  Add_9f284 : Sum
  Add_afd7a : Sum
  Constant_-1_3ecb0 : Constant  Value=-1
  Product_8c49f : Product
  Blockout_id_bus_20_0c62a : Outport
  wires:
  State_id_line_10_20_7e98a/1 -> Add_9f284/2
  Product_8c49f/1 -> Add_9f284/1
  State_id_load_20_3e20a/1 -> Product_8c49f/2
  Constant_-1_3ecb0/1 -> Product_8c49f/1
  Add_9f284/1 -> Add_afd7a/1
  State_id_line_19_20_ee948/1 -> Add_afd7a/2
  Add_afd7a/1 -> Blockout_id_bus_20_0c62a/1

== system IEEE30_case/AC_1/id_bus_21_block ==
  note: id_bus_21 in IEEE30_case
      | $\mathrm{id}_{\mathrm{line},10,21}-\mathrm{id}_{\mathrm{load},21}-\mathrm{id}_{\mathrm{line},21,22}$
      | Automatically generated on 2025-11-01 18:43:10 .
  State_id_load_21_b42be : Inport
  State_id_line_10_21_bcd00 : Inport  Port=2
  State_id_line_21_22_cc9c2 : Inport  Port=3
  Add_f1bd6 : Sum
  Constant_-1_f9414 : Constant  Value=-1
  Product_16f61 : Product
  Subtract_cc501 : Sum  Inputs=+-
  Blockout_id_bus_21_f6b53 : Outport
  wires:
  Subtract_cc501/1 -> Blockout_id_bus_21_f6b53/1
  Product_16f61/1 -> Add_f1bd6/1
  Constant_-1_f9414/1 -> Product_16f61/1
  Add_f1bd6/1 -> Subtract_cc501/1
  State_id_line_10_21_bcd00/1 -> Add_f1bd6/2
  State_id_load_21_b42be/1 -> Product_16f61/2
  State_id_line_21_22_cc9c2/1 -> Subtract_cc501/2

== system IEEE30_case/AC_1/id_bus_22_block ==
  note: id_bus_22 in IEEE30_case
      | $\mathrm{id}_{\mathrm{SG},D,22}+\mathrm{id}_{\mathrm{line},10,22}+\mathrm{id}_{\mathrm{line},21,22}-\mathrm{id}_{\mathrm{line},22,24}$
      | Automatically generated on 2025-11-01 18:43:13 .
  Input_id_SG_D_22_c72e9 : Inport
  State_id_line_10_22_83f91 : Inport  Port=2
  State_id_line_21_22_cc6ca : Inport  Port=3
  State_id_line_22_24_1a6a9 : Inport  Port=4
  Add_461c8 : Sum
  Add_acbc8 : Sum
  Subtract_f1aad : Sum  Inputs=+-
  Blockout_id_bus_22_34fe4 : Outport
  wires:
  Add_461c8/1 -> Add_acbc8/1
  Input_id_SG_D_22_c72e9/1 -> Add_461c8/1
  State_id_line_10_22_83f91/1 -> Add_461c8/2
  State_id_line_22_24_1a6a9/1 -> Subtract_f1aad/2
  State_id_line_21_22_cc6ca/1 -> Add_acbc8/2
  Subtract_f1aad/1 -> Blockout_id_bus_22_34fe4/1
  Add_acbc8/1 -> Subtract_f1aad/1

== system IEEE30_case/AC_1/id_bus_23_block ==
  note: id_bus_23 in IEEE30_case
      | $\mathrm{id}_{\mathrm{SG},D,23}-\mathrm{id}_{\mathrm{load},23}+\mathrm{id}_{\mathrm{line},15,23}-\mathrm{id}_{\mathrm{line},23,24}$
      | Automatically generated on 2025-11-01 18:43:17 .
  Input_id_SG_D_23_b9b6b : Inport
  State_id_load_23_5361b : Inport  Port=2
  State_id_line_15_23_e01a5 : Inport  Port=3
  State_id_line_23_24_0bbc7 : Inport  Port=4
  Add_f0824 : Sum
  Subtract_3f692 : Sum  Inputs=+-
  Subtract_a2e65 : Sum  Inputs=+-
  Blockout_id_bus_23_84113 : Outport
  wires:
  Subtract_3f692/1 -> Add_f0824/1
  Input_id_SG_D_23_b9b6b/1 -> Subtract_3f692/1
  Add_f0824/1 -> Subtract_a2e65/1
  State_id_load_23_5361b/1 -> Subtract_3f692/2
  State_id_line_15_23_e01a5/1 -> Add_f0824/2
  State_id_line_23_24_0bbc7/1 -> Subtract_a2e65/2
  Subtract_a2e65/1 -> Blockout_id_bus_23_84113/1

== system IEEE30_case/AC_1/id_bus_24_block ==
  note: id_bus_24 in IEEE30_case
      | $\mathrm{id}_{\mathrm{line},22,24}-\mathrm{id}_{\mathrm{load},24}+\mathrm{id}_{\mathrm{line},23,24}-\mathrm{id}_{\mathrm{line},24,25}$
      | Automatically generated on 2025-11-01 18:43:18 .
  State_id_load_24_1483c : Inport
  State_id_line_22_24_03003 : Inport  Port=2
  State_id_line_23_24_8269a : Inport  Port=3
  State_id_line_24_25_6b48d : Inport  Port=4
  Add_6b3d2 : Sum
  Add_feefa : Sum
  Constant_-1_cd638 : Constant  Value=-1
  Product_1ead9 : Product
  Subtract_d3e9b : Sum  Inputs=+-
  Blockout_id_bus_24_85e6b : Outport
  wires:
  State_id_line_24_25_6b48d/1 -> Subtract_d3e9b/2
  Constant_-1_cd638/1 -> Product_1ead9/1
  Product_1ead9/1 -> Add_feefa/1
  Add_feefa/1 -> Add_6b3d2/1
  Add_6b3d2/1 -> Subtract_d3e9b/1
  State_id_line_22_24_03003/1 -> Add_feefa/2
  State_id_load_24_1483c/1 -> Product_1ead9/2
  State_id_line_23_24_8269a/1 -> Add_6b3d2/2
  Subtract_d3e9b/1 -> Blockout_id_bus_24_85e6b/1

== system IEEE30_case/AC_1/id_bus_25_block ==
  note: id_bus_25 in IEEE30_case
      | $\mathrm{id}_{\mathrm{line},24,25}-\mathrm{id}_{\mathrm{line},25,26}-\mathrm{id}_{\mathrm{line},25,27}$
      | Automatically generated on 2025-11-01 18:43:20 .
  State_id_line_24_25_2e897 : Inport
  State_id_line_25_26_94c65 : Inport  Port=2
  State_id_line_25_27_89c78 : Inport  Port=3
  Subtract_10cd1 : Sum  Inputs=+-
  Subtract_2e0f9 : Sum  Inputs=+-
  Blockout_id_bus_25_a9e73 : Outport
  wires:
  State_id_line_24_25_2e897/1 -> Subtract_10cd1/1
  State_id_line_25_26_94c65/1 -> Subtract_10cd1/2
  Subtract_10cd1/1 -> Subtract_2e0f9/1
  State_id_line_25_27_89c78/1 -> Subtract_2e0f9/2
  Subtract_2e0f9/1 -> Blockout_id_bus_25_a9e73/1

== system IEEE30_case/AC_1/id_bus_26_block ==
  note: id_bus_26 in IEEE30_case
      | $\mathrm{id}_{\mathrm{line},25,26}-\mathrm{id}_{\mathrm{load},26}$
      | Automatically generated on 2025-11-01 18:43:21 .
  State_id_load_26_80bb7 : Inport
  State_id_line_25_26_45789 : Inport  Port=2
  Add_73153 : Sum
  Constant_-1_d2ca6 : Constant  Value=-1
  Product_65519 : Product
  Blockout_id_bus_26_f258d : Outport
  wires:
  State_id_line_25_26_45789/1 -> Add_73153/2
  State_id_load_26_80bb7/1 -> Product_65519/2
  Constant_-1_d2ca6/1 -> Product_65519/1
  Product_65519/1 -> Add_73153/1
  Add_73153/1 -> Blockout_id_bus_26_f258d/1

== system IEEE30_case/AC_1/id_bus_27_block ==
  note: id_bus_27 in IEEE30_case
      | $\mathrm{id}_{\mathrm{SG},D,27}+\mathrm{id}_{\mathrm{line},25,27}-\mathrm{id}_{\mathrm{line},27,29}-\mathrm{id}_{\mathrm{line},27,30}+\mathrm{id}_{\mathrm{line},28,27}$
      | Automatically generated on 2025-11-01 18:43:24 .
  Input_id_SG_D_27_bfa21 : Inport
  State_id_line_25_27_a3c54 : Inport  Port=2
  State_id_line_27_29_ed62c : Inport  Port=3
  State_id_line_27_30_1b75b : Inport  Port=4
  State_id_line_28_27_22b40 : Inport  Port=5
  Add_4be4a : Sum
  Add_fdb23 : Sum
  Subtract_05e48 : Sum  Inputs=+-
  Subtract_ddc00 : Sum  Inputs=+-
  Blockout_id_bus_27_09b01 : Outport
  wires:
  Input_id_SG_D_27_bfa21/1 -> Add_fdb23/1
  Add_fdb23/1 -> Subtract_ddc00/1
  State_id_line_27_30_1b75b/1 -> Subtract_05e48/2
  State_id_line_25_27_a3c54/1 -> Add_fdb23/2
  State_id_line_27_29_ed62c/1 -> Subtract_ddc00/2
  Subtract_ddc00/1 -> Subtract_05e48/1
  Subtract_05e48/1 -> Add_4be4a/1
  State_id_line_28_27_22b40/1 -> Add_4be4a/2
  Add_4be4a/1 -> Blockout_id_bus_27_09b01/1

== system IEEE30_case/AC_1/id_bus_28_block ==
  note: id_bus_28 in IEEE30_case
      | $\mathrm{id}_{\mathrm{line},6,28}+\mathrm{id}_{\mathrm{line},8,28}-\mathrm{id}_{\mathrm{line},28,27}$
      | Automatically generated on 2025-11-01 18:43:26 .
  State_id_line_6_28_b8533 : Inport
  State_id_line_8_28_46f95 : Inport  Port=2
  State_id_line_28_27_48f21 : Inport  Port=3
  Add_a5c1b : Sum
  Subtract_24494 : Sum  Inputs=+-
  Blockout_id_bus_28_5bbbe : Outport
  wires:
  State_id_line_6_28_b8533/1 -> Add_a5c1b/1
  State_id_line_8_28_46f95/1 -> Add_a5c1b/2
  Add_a5c1b/1 -> Subtract_24494/1
  State_id_line_28_27_48f21/1 -> Subtract_24494/2
  Subtract_24494/1 -> Blockout_id_bus_28_5bbbe/1

== system IEEE30_case/AC_1/id_bus_29_block ==
  note: id_bus_29 in IEEE30_case
      | $\mathrm{id}_{\mathrm{line},27,29}-\mathrm{id}_{\mathrm{load},29}-\mathrm{id}_{\mathrm{line},29,30}$
      | Automatically generated on 2025-11-01 18:43:27 .
  State_id_load_29_01b75 : Inport
  State_id_line_27_29_0ffe7 : Inport  Port=2
  State_id_line_29_30_80eff : Inport  Port=3
  Add_e3f6b : Sum
  Constant_-1_c2df0 : Constant  Value=-1
  Product_5604d : Product
  Subtract_832d2 : Sum  Inputs=+-
  Blockout_id_bus_29_dcea9 : Outport
  wires:
  Subtract_832d2/1 -> Blockout_id_bus_29_dcea9/1
  Constant_-1_c2df0/1 -> Product_5604d/1
  Product_5604d/1 -> Add_e3f6b/1
  State_id_load_29_01b75/1 -> Product_5604d/2
  State_id_line_29_30_80eff/1 -> Subtract_832d2/2
  State_id_line_27_29_0ffe7/1 -> Add_e3f6b/2
  Add_e3f6b/1 -> Subtract_832d2/1

== system IEEE30_case/AC_1/id_bus_2_block ==
  note: id_bus_2 in IEEE30_case
      | $\mathrm{id}_{\mathrm{SG},D,2}-\mathrm{id}_{\mathrm{load},2}+\mathrm{id}_{\mathrm{line},1,2}-\mathrm{id}_{\mathrm{line},2,4}-\mathrm{id}_{\mathrm{line},2,5}-\mathrm{id}_{\mathrm{line},2,6}$
      | Automatically generated on 2025-11-01 18:42:36 .
  Input_id_SG_D_2_271b9 : Inport
  State_id_load_2_17a4a : Inport  Port=2
  State_id_line_1_2_35b9f : Inport  Port=3
  State_id_line_2_4_9c9be : Inport  Port=4
  State_id_line_2_5_1281e : Inport  Port=5
  State_id_line_2_6_b437f : Inport  Port=6
  Add_f22ec : Sum
  Subtract_02f60 : Sum  Inputs=+-
  Subtract_42936 : Sum  Inputs=+-
  Subtract_a5b4e : Sum  Inputs=+-
  Subtract_b4c90 : Sum  Inputs=+-
  Blockout_id_bus_2_bbec8 : Outport
  wires:
  Input_id_SG_D_2_271b9/1 -> Subtract_b4c90/1
  Subtract_b4c90/1 -> Add_f22ec/1
  State_id_line_1_2_35b9f/1 -> Add_f22ec/2
  State_id_load_2_17a4a/1 -> Subtract_b4c90/2
  Add_f22ec/1 -> Subtract_02f60/1
  Subtract_02f60/1 -> Subtract_42936/1
  State_id_line_2_4_9c9be/1 -> Subtract_02f60/2
  State_id_line_2_5_1281e/1 -> Subtract_42936/2
  Subtract_42936/1 -> Subtract_a5b4e/1
  State_id_line_2_6_b437f/1 -> Subtract_a5b4e/2
  Subtract_a5b4e/1 -> Blockout_id_bus_2_bbec8/1

== system IEEE30_case/AC_1/id_bus_30_block ==
  note: id_bus_30 in IEEE30_case
      | $\mathrm{id}_{\mathrm{line},27,30}-\mathrm{id}_{\mathrm{load},30}+\mathrm{id}_{\mathrm{line},29,30}$
      | Automatically generated on 2025-11-01 18:43:29 .
  State_id_load_30_9a1a0 : Inport
  State_id_line_27_30_55115 : Inport  Port=2
  State_id_line_29_30_b478a : Inport  Port=3
  Add_21e0a : Sum
  Add_4ee42 : Sum
  Constant_-1_10703 : Constant  Value=-1
  Product_0316f : Product
  Blockout_id_bus_30_50341 : Outport
  wires:
  Add_21e0a/1 -> Blockout_id_bus_30_50341/1
  Product_0316f/1 -> Add_4ee42/1
  Constant_-1_10703/1 -> Product_0316f/1
  State_id_line_27_30_55115/1 -> Add_4ee42/2
  State_id_load_30_9a1a0/1 -> Product_0316f/2
  Add_4ee42/1 -> Add_21e0a/1
  State_id_line_29_30_b478a/1 -> Add_21e0a/2

== system IEEE30_case/AC_1/id_bus_3_block ==
  note: id_bus_3 in IEEE30_case
      | $\mathrm{id}_{\mathrm{line},1,3}-\mathrm{id}_{\mathrm{load},3}-\mathrm{id}_{\mathrm{line},3,4}$
      | Automatically generated on 2025-11-01 18:42:37 .
  State_id_load_3_6a44d : Inport
  State_id_line_1_3_85a3c : Inport  Port=2
  State_id_line_3_4_6ece1 : Inport  Port=3
  Add_68df8 : Sum
  Constant_-1_ae9aa : Constant  Value=-1
  Product_f4fb2 : Product
  Subtract_3196e : Sum  Inputs=+-
  Blockout_id_bus_3_36e80 : Outport
  wires:
  Subtract_3196e/1 -> Blockout_id_bus_3_36e80/1
  Constant_-1_ae9aa/1 -> Product_f4fb2/1
  State_id_load_3_6a44d/1 -> Product_f4fb2/2
  Product_f4fb2/1 -> Add_68df8/1
  State_id_line_3_4_6ece1/1 -> Subtract_3196e/2
  State_id_line_1_3_85a3c/1 -> Add_68df8/2
  Add_68df8/1 -> Subtract_3196e/1

== system IEEE30_case/AC_1/id_bus_4_block ==
  note: id_bus_4 in IEEE30_case
      | $\mathrm{id}_{\mathrm{line},2,4}-\mathrm{id}_{\mathrm{load},4}+\mathrm{id}_{\mathrm{line},3,4}-\mathrm{id}_{\mathrm{line},4,6}-\mathrm{id}_{\mathrm{line},4,12}$
      | Automatically generated on 2025-11-01 18:42:39 .
  State_id_load_4_57c3e : Inport
  State_id_line_2_4_e4641 : Inport  Port=2
  State_id_line_3_4_41268 : Inport  Port=3
  State_id_line_4_6_c02d6 : Inport  Port=4
  State_id_line_4_12_0ad5f : Inport  Port=5
  Add_45dd3 : Sum
  Add_6cee2 : Sum
  Constant_-1_d995f : Constant  Value=-1
  Product_7d985 : Product
  Subtract_6739f : Sum  Inputs=+-
  Subtract_7cda2 : Sum  Inputs=+-
  Blockout_id_bus_4_62c4e : Outport
  wires:
  State_id_line_4_6_c02d6/1 -> Subtract_6739f/2
  Constant_-1_d995f/1 -> Product_7d985/1
  Product_7d985/1 -> Add_45dd3/1
  Add_45dd3/1 -> Add_6cee2/1
  State_id_line_2_4_e4641/1 -> Add_45dd3/2
  State_id_load_4_57c3e/1 -> Product_7d985/2
  State_id_line_3_4_41268/1 -> Add_6cee2/2
  Add_6cee2/1 -> Subtract_6739f/1
  Subtract_6739f/1 -> Subtract_7cda2/1
  State_id_line_4_12_0ad5f/1 -> Subtract_7cda2/2
  Subtract_7cda2/1 -> Blockout_id_bus_4_62c4e/1

== system IEEE30_case/AC_1/id_bus_5_block ==
  note: id_bus_5 in IEEE30_case
      | $\mathrm{id}_{\mathrm{line},2,5}-\mathrm{id}_{\mathrm{line},5,7}$
      | Automatically generated on 2025-11-01 18:42:41 .
  State_id_line_2_5_9c966 : Inport
  State_id_line_5_7_98a48 : Inport  Port=2
  Subtract_a9f1d : Sum  Inputs=+-
  Blockout_id_bus_5_f0a59 : Outport
  wires:
  State_id_line_2_5_9c966/1 -> Subtract_a9f1d/1
  State_id_line_5_7_98a48/1 -> Subtract_a9f1d/2
  Subtract_a9f1d/1 -> Blockout_id_bus_5_f0a59/1

== system IEEE30_case/AC_1/id_bus_6_block ==
  note: id_bus_6 in IEEE30_case
      | $\mathrm{id}_{\mathrm{line},2,6}+\mathrm{id}_{\mathrm{line},4,6}-\mathrm{id}_{\mathrm{line},6,7}-\mathrm{id}_{\mathrm{line},6,8}-\mathrm{id}_{\mathrm{line},6,9}-\mathrm{id}_{\mathrm{line},6,10}-\mathrm{id}_{\mathrm{line},6,28}$
      | Automatically generated on 2025-11-01 18:42:42 .
  State_id_line_2_6_f1c81 : Inport
  State_id_line_4_6_eeef8 : Inport  Port=2
  State_id_line_6_7_6920a : Inport  Port=3
  State_id_line_6_8_8d48d : Inport  Port=4
  State_id_line_6_9_c95db : Inport  Port=5
  State_id_line_6_10_2c687 : Inport  Port=6
  State_id_line_6_28_5760f : Inport  Port=7
  Add_f8d28 : Sum
  Subtract_20e5a : Sum  Inputs=+-
  Subtract_4fb67 : Sum  Inputs=+-
  Subtract_57b90 : Sum  Inputs=+-
  Subtract_92b6e : Sum  Inputs=+-
  Subtract_c26e8 : Sum  Inputs=+-
  Blockout_id_bus_6_41f21 : Outport
  wires:
  State_id_line_2_6_f1c81/1 -> Add_f8d28/1
  State_id_line_4_6_eeef8/1 -> Add_f8d28/2
  Add_f8d28/1 -> Subtract_92b6e/1
  Subtract_92b6e/1 -> Subtract_20e5a/1
  State_id_line_6_8_8d48d/1 -> Subtract_20e5a/2
  State_id_line_6_7_6920a/1 -> Subtract_92b6e/2
  Subtract_57b90/1 -> Subtract_4fb67/1
  Subtract_20e5a/1 -> Subtract_57b90/1
  State_id_line_6_9_c95db/1 -> Subtract_57b90/2
  State_id_line_6_10_2c687/1 -> Subtract_4fb67/2
  Subtract_c26e8/1 -> Blockout_id_bus_6_41f21/1
  Subtract_4fb67/1 -> Subtract_c26e8/1
  State_id_line_6_28_5760f/1 -> Subtract_c26e8/2

== system IEEE30_case/AC_1/id_bus_7_block ==
  note: id_bus_7 in IEEE30_case
      | $\mathrm{id}_{\mathrm{line},5,7}-\mathrm{id}_{\mathrm{load},7}+\mathrm{id}_{\mathrm{line},6,7}+\mathrm{id}_{\mathrm{GFL},\mathrm{DFIG},7}$
      | Automatically generated on 2025-11-01 18:42:46 .
  Input_id_GFL_DFIG_7_848f8 : Inport
  State_id_load_7_78ca4 : Inport  Port=2
  State_id_line_5_7_86c29 : Inport  Port=3
  State_id_line_6_7_ce94d : Inport  Port=4
  Add_f6d18 : Sum
  Add_fa306 : Sum
  Subtract_1fe25 : Sum  Inputs=+-
  Blockout_id_bus_7_1a1e5 : Outport
  wires:
  Subtract_1fe25/1 -> Add_f6d18/1
  Input_id_GFL_DFIG_7_848f8/1 -> Subtract_1fe25/1
  State_id_load_7_78ca4/1 -> Subtract_1fe25/2
  State_id_line_6_7_ce94d/1 -> Add_fa306/2
  State_id_line_5_7_86c29/1 -> Add_f6d18/2
  Add_fa306/1 -> Blockout_id_bus_7_1a1e5/1
  Add_f6d18/1 -> Add_fa306/1

== system IEEE30_case/AC_1/id_bus_8_block ==
  note: id_bus_8 in IEEE30_case
      | $\mathrm{id}_{\mathrm{line},6,8}-\mathrm{id}_{\mathrm{load},8}-\mathrm{id}_{\mathrm{line},8,28}$
      | Automatically generated on 2025-11-01 18:42:47 .
  State_id_load_8_2d300 : Inport
  State_id_line_6_8_e60f9 : Inport  Port=2
  State_id_line_8_28_28354 : Inport  Port=3
  Add_ee3b1 : Sum
  Constant_-1_65cca : Constant  Value=-1
  Product_04f98 : Product
  Subtract_bb07f : Sum  Inputs=+-
  Blockout_id_bus_8_ac02c : Outport
  wires:
  Subtract_bb07f/1 -> Blockout_id_bus_8_ac02c/1
  Product_04f98/1 -> Add_ee3b1/1
  Constant_-1_65cca/1 -> Product_04f98/1
  State_id_line_6_8_e60f9/1 -> Add_ee3b1/2
  State_id_load_8_2d300/1 -> Product_04f98/2
  Add_ee3b1/1 -> Subtract_bb07f/1
  State_id_line_8_28_28354/1 -> Subtract_bb07f/2

== system IEEE30_case/AC_1/id_bus_9_block ==
  note: id_bus_9 in IEEE30_case
      | $\mathrm{id}_{\mathrm{line},6,9}-\mathrm{id}_{\mathrm{line},9,10}-\mathrm{id}_{\mathrm{line},9,11}$
      | Automatically generated on 2025-11-01 18:42:49 .
  State_id_line_6_9_06348 : Inport
  State_id_line_9_10_f038a : Inport  Port=2
  State_id_line_9_11_17709 : Inport  Port=3
  Subtract_2b4e7 : Sum  Inputs=+-
  Subtract_605fe : Sum  Inputs=+-
  Blockout_id_bus_9_0b36c : Outport
  wires:
  State_id_line_9_11_17709/1 -> Subtract_605fe/2
  State_id_line_6_9_06348/1 -> Subtract_2b4e7/1
  State_id_line_9_10_f038a/1 -> Subtract_2b4e7/2
  Subtract_2b4e7/1 -> Subtract_605fe/1
  Subtract_605fe/1 -> Blockout_id_bus_9_0b36c/1

== system IEEE30_case/AC_1/iq_bus_10_block ==
  note: iq_bus_10 in IEEE30_case
      | $\mathrm{iq}_{\mathrm{line},6,10}-\mathrm{iq}_{\mathrm{load},10}+\mathrm{iq}_{\mathrm{line},9,10}-\mathrm{iq}_{\mathrm{line},10,17}-\mathrm{iq}_{\mathrm{line},10,20}-\mathrm{iq}_{\mathrm{line},10,21}-\mathrm{iq}_{\mathrm{line},10,22}$
      | Automatically generated on 2025-11-01 18:42:52 .
  State_iq_load_10_2c7ec : Inport
  State_iq_line_6_10_9ea7c : Inport  Port=2
  State_iq_line_9_10_547ec : Inport  Port=3
  State_iq_line_10_17_d7997 : Inport  Port=4
  State_iq_line_10_20_d3f34 : Inport  Port=5
  State_iq_line_10_21_f5701 : Inport  Port=6
  State_iq_line_10_22_b2379 : Inport  Port=7
  Add_a5e0a : Sum
  Add_f5ab7 : Sum
  Constant_-1_9c0b9 : Constant  Value=-1
  Product_29c30 : Product
  Subtract_69cfa : Sum  Inputs=+-
  Subtract_a840e : Sum  Inputs=+-
  Subtract_b575a : Sum  Inputs=+-
  Subtract_da2cb : Sum  Inputs=+-
  Blockout_iq_bus_10_f080b : Outport
  wires:
  Constant_-1_9c0b9/1 -> Product_29c30/1
  Product_29c30/1 -> Add_f5ab7/1
  State_iq_load_10_2c7ec/1 -> Product_29c30/2
  State_iq_line_9_10_547ec/1 -> Add_a5e0a/2
  State_iq_line_6_10_9ea7c/1 -> Add_f5ab7/2
  Add_f5ab7/1 -> Add_a5e0a/1
  Add_a5e0a/1 -> Subtract_da2cb/1
  State_iq_line_10_17_d7997/1 -> Subtract_da2cb/2
  Subtract_da2cb/1 -> Subtract_69cfa/1
  State_iq_line_10_20_d3f34/1 -> Subtract_69cfa/2
  Subtract_69cfa/1 -> Subtract_a840e/1
  State_iq_line_10_21_f5701/1 -> Subtract_a840e/2
  Subtract_a840e/1 -> Subtract_b575a/1
  State_iq_line_10_22_b2379/1 -> Subtract_b575a/2
  Subtract_b575a/1 -> Blockout_iq_bus_10_f080b/1

== system IEEE30_case/AC_1/iq_bus_11_block ==
  note: iq_bus_11 in IEEE30_case
      | $\mathrm{iq}_{\mathrm{line},9,11}$
      | Automatically generated on 2025-11-01 18:42:53 .
  State_iq_line_9_11_5dafe : Inport
  Blockout_iq_bus_11_40b0f : Outport
  wires:
  State_iq_line_9_11_5dafe/1 -> Blockout_iq_bus_11_40b0f/1
